simulink model "WindPrototipeN"  (R2019b)
settings: Solver=ode23s  StartTime=0.0  StopTime=Ts  FixedStep=2  RelTol=5
values from neighbouring files (symbols this model uses):
  c1 = 0.51763    [matlab.mat]
  c2 = 116    [matlab.mat]
  c3 = 0.4    [matlab.mat]
  c4 = 5    [matlab.mat]
  c5 = 21    [matlab.mat]
  c6 = 0.006795    [matlab.mat]
  Tp = 2e-05    [matlab.mat]
undefined symbols (not defined in the file or in its folder): Cogent, DiscIntNeverNeededParam, Ion, Kepware, Lithium, localhost, sigbuilder_block
libraries: powerlib x266, powerlib_extras x83, simulink x30, powerlib_meascontrol x13, opclib x11, sldrtlib x8, electricdrivelib x3
(part 5 of 9)

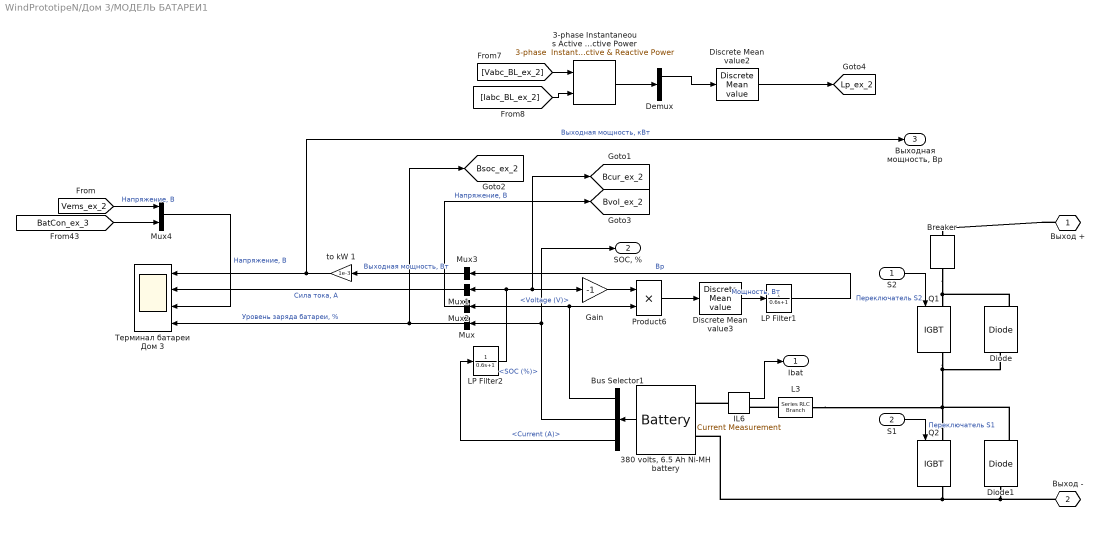
== system WindPrototipeN/Дом 3/МОДЕЛЬ БАТАРЕИ1 ==
  S2 : Inport
  S1 : Inport  Port=2
  3-phase Instantaneous Active & Reactive Power : powerlib_extras/Measurements/3-phase  Instantaneous  Active & Reactive Power
      settings: SourceProductName=Simscape Electrical  SourceProductBaseCode=PS
  "380 volts, 6.5 Ah Ni-MH battery " : electricdrivelib/Extra Sources/Battery  BatType=Lithium-Ion  ShowTempParam=off  ThermalPreset=no  ShowAgeParam=off  NomV=380  NomQ=2  SOC=56  Batt_Tr=10  PresetModel=on  MaxQ=2  MinV=285  FullV=442.3151  Dis_rate=0.86957  R=1.9  Normal_OP=1.8087  expZone="[410.5466    0.09826087]"  current=[6.5 13 32.5]  Units=Time  Tci=20  NomT=20  T2=-30  MaxQ2=4.8  FullV2=7.1  Normal_OP2=5.655  expZone2="[6.58           1]"  Rca=0.6  ti=2000  Dp=0  Neq0=0  Tsim=1e6  Ta1=25  Qeol=5.4*0.9  Reol=0.013333*1.2  Char_age=[2.3478, 3]  Dis_age=[2.3478, 10]  N1=1500  N2=10500  N3=1000  N4=1400  Ta2=45  N5=950
      settings: SourceProductName=Simscape Electrical
  Breaker : powerlib/Elements/Breaker  InitialState=1  SwitchingTimes=[15 ]  External=off  BreakerResistance=0.01  SnubberResistance=1e6  SnubberCapacitance=inf  Measurements=None  MoreParameters=off  NoBreakLoop=off
      settings: SourceProductName=Simscape Electrical
  Bus Selector1 : BusSelector  OutputSignals=Voltage (V),SOC (%),Current (A)
  Demux : Demux  Outputs=2
  Diode : powerlib/Power Electronics/Diode  Ron=0.001  Lon=0  Vf=0.8  IC=0  UseSnubber=off  Rs=500  Cs=250e-9  Measurements=on
      settings: SourceProductName=Simscape Electrical
  Diode1 : powerlib/Power Electronics/Diode  Ron=0.001  Lon=0  Vf=0.8  IC=0  UseSnubber=off  Rs=500  Cs=250e-9  Measurements=on
      settings: SourceProductName=Simscape Electrical
  Discrete Mean value2 : powerlib_extras/Discrete Measurements/Discrete  Mean value  Freq=50  Vinit=0  Ts=20e-6
      settings: SourceProductName=Simscape Electrical  SourceProductBaseCode=PS
  Discrete Mean value3 : powerlib_extras/Discrete Measurements/Discrete  Mean value  Freq=50  Vinit=0  Ts=20e-6
      settings: SourceProductName=Simscape Electrical  SourceProductBaseCode=PS
  Gain : Gain  Gain=-1
  IL6 : powerlib/Measurements/Current Measurement  PhasorSimulation=off  OutputType=Complex  PSBequivalent=0
      settings: SourceProductName=Simscape Electrical
  L3 : powerlib/Elements/Series RLC Branch  LConnTagsString=__new0  RConnTagsString=__new0  BranchType=L  Resistance=1.0  Inductance=5e-3  SetiL0=off  InitialCurrent=0  Capacitance=1.0  Setx0=off  InitialVoltage=0  Measurements=None
      settings: SourceProductName=Simscape Electrical
  LP Filter1 : TransferFcn  Denominator=[0.6 1]
  LP Filter2 : TransferFcn  Denominator=[0.6 1]
  Mux{,1..3} (4 alike) : Mux  Inputs=1
  Mux4 : Mux  Inputs=2
  Product6 : Product  RndMeth=Zero
  Q1 : powerlib/Power Electronics/IGBT  Ron=0.001  Lon=0  Vf=1  Tf=1e-6  Tt=2e-6  IC=0  Rs=1e5  Cs=inf  Measurements=on
      settings: SourceProductName=Simscape Electrical
  Q2 : powerlib/Power Electronics/IGBT  Ron=0.001  Lon=0  Vf=1  Tf=1e-6  Tt=2e-6  IC=0  Rs=1e5  Cs=inf  Measurements=on
      settings: SourceProductName=Simscape Electrical
  to kW 1 : Gain  Gain=1e-3
  Терминал батареи Дом 3 : Scope  NumInputPorts=4
  Выход + : PMIOPort  Tag=PMCPort  Side=Right
  " Выход -" : PMIOPort  Tag=PMCPort  Port=2  Side=Right
  Ibat : Outport  VectorParamsAs1DForOutWhenUnconnected=off
  "SOC, %" : Outport  Port=2  VectorParamsAs1DForOutWhenUnconnected=off
  "Выходная мощность, Bp" : Outport  Port=3  VectorParamsAs1DForOutWhenUnconnected=off
  tag scope: Bcur_ex_2=global, Bsoc_ex_2=global, Bvol_ex_2=global, Lp_ex_2=global
  wires:
  "380 volts, 6.5 Ah Ni-MH battery "/1 -> Bus Selector1/1
  Bus Selector1/1 -> Mux2/1, Product6/2  "<Voltage (V)>"
  Bus Selector1/2 -> Mux/1, "SOC, %"/1  "<SOC (%)>"
  Bus Selector1/3 -> LP Filter2/1  "<Current (A)>"
  S2/1 -> Q1/1  "Переключатель S2"
  S1/1 -> Q2/1  "Переключатель S1"
  IL6/1 -> Ibat/1
  Gain/1 -> Product6/1
  LP Filter2/1 -> Mux1/1, [Bcur_ex_2], Gain/1
  Discrete Mean value3/1 -> LP Filter1/1  "Мощность, Вт"
  Mux/1 -> [Bsoc_ex_2], Терминал батареи Дом 3/4  "Уровень заряда батареи, %"
  Mux1/1 -> Терминал батареи Дом 3/2  "Сила тока, А"
  Mux3/1 -> to kW 1/1  "Выходная мощность, Вт"
  Product6/1 -> Discrete Mean value3/1
  [Iabc_BL_ex_2] -> 3-phase Instantaneous Active & Reactive Power/2
  Discrete Mean value2/1 -> [Lp_ex_2]
  [Vabc_BL_ex_2] -> 3-phase Instantaneous Active & Reactive Power/1
  to kW 1/1 -> "Выходная мощность, Bp"/1, Терминал батареи Дом 3/1  "Выходная мощность, кВт"
  LP Filter1/1 -> Mux3/1  "Bp"
  Demux/1 -> Discrete Mean value2/1
  3-phase Instantaneous Active & Reactive Power/1 -> Demux/1
  Mux2/1 -> [Bvol_ex_2]  "Напряжение, В"
  [Vems_ex_2] -> Mux4/1  "Напряжение, В"
  Mux4/1 -> Терминал батареи Дом 3/3  "Напряжение, В"
  [BatCon_ex_3] -> Mux4/2
  connections:
  IL6/LConn1 -- "380 volts, 6.5 Ah Ni-MH battery "/LConn1
  Q2/RConn1 -- " Выход -"/RConn1 -- Diode1/LConn1 -- "380 volts, 6.5 Ah Ni-MH battery "/LConn2
  Выход +/RConn1 -- Breaker/LConn1
  Breaker/RConn1 -- Diode/RConn1 -- Q1/LConn1
  Q2/LConn1 -- Diode1/RConn1 -- Q1/RConn1 -- Diode/LConn1 -- L3/RConn1
  L3/LConn1 -- IL6/RConn1

== system WindPrototipeN/Дом 3/Мониторинг мощностей ==
  " to kW1" : Gain  Gain=1e-3
  Bus Creator1 : BusCreator  Inputs=4
  Discrete Mean value2 : powerlib_extras/Discrete Measurements/Discrete  Mean value  Freq=50  Vinit=0  Ts=20e-6
      settings: SourceProductName=Simscape Electrical  SourceProductBaseCode=PS
  Discrete Mean value3 : powerlib_extras/Discrete Measurements/Discrete  Mean value  Freq=50  Vinit=0  Ts=20e-6
      settings: SourceProductName=Simscape Electrical  SourceProductBaseCode=PS
  Discrete Mean value4 : powerlib_extras/Discrete Measurements/Discrete  Mean value  Freq=50  Vinit=0  Ts=20e-6
      settings: SourceProductName=Simscape Electrical  SourceProductBaseCode=PS
  "Power (3ph, Phasor)2" : powerlib_meascontrol/Measurements/Power (3ph, Phasor)
      settings: SourceProductName=Simscape Electrical  SourceProductBaseCode=PS
  Terminator2 : Terminator
  to kW 1 : Gain  Gain=1e-3
  to kW 2 : Gain  Gain=1e-3
  to kW 4 : Gain  Gain=1e-3
  Мощности Дом 3 : Scope
  wires:
  [Vload_ex_2] -> "Power (3ph, Phasor)2"/1
  [Lp_ex_2] -> to kW 1/1  "LP"
  [Wp_ex_2] -> Discrete Mean value4/1
  "Power (3ph, Phasor)2"/2 -> Terminator2/1
  Discrete Mean value2/1 -> " to kW1"/1
  to kW 2/1 -> Bus Creator1/3  "WP"
  to kW 4/1 -> Bus Creator1/2  "SP"
  " to kW1"/1 -> Bus Creator1/4  "Нагрузка"
  Discrete Mean value4/1 -> to kW 2/1
  [Iload_ex_2] -> "Power (3ph, Phasor)2"/2
  "Power (3ph, Phasor)2"/1 -> Discrete Mean value2/1
  Bus Creator1/1 -> Мощности Дом 3/1
  [Sp_ex_2] -> Discrete Mean value3/1
  Discrete Mean value3/1 -> to kW 4/1
  to kW 1/1 -> Bus Creator1/1  "Реактивная Б-Н"

== system WindPrototipeN/Дом 3/ПОТРЕБИТЕЛЬ1 ==
  1000 Вт1 : powerlib/Elements/Three-Phase Parallel RLC Load  LConnTagsString=A|B|C  Configuration=Y (grounded)  NominalVoltage=385  Vabc=[1e3 1e3 1e3]  Vabcp=[1e3 1e3 1e3]  NominalFrequency=50  UnbalancedPower=off  ActivePower=1000  InductivePower=0  CapacitivePower=0  Pabc=[10e3 9e3 11e3]  QLabc=[100 90 110]  QCabc=[100 90 110]  Pabcp=[10e3 9e3 11e3]  QLabcp=[100 90 110]  QCabcp=[100 90 110]  Measurements=None  LoadType=constant Z
      settings: SourceProductName=Simscape Electrical
  1500 Вт1 : powerlib/Elements/Three-Phase Parallel RLC Load  LConnTagsString=A|B|C  Configuration=Y (grounded)  NominalVoltage=385  Vabc=[1e3 1e3 1e3]  Vabcp=[1e3 1e3 1e3]  NominalFrequency=50  UnbalancedPower=off  ActivePower=1000  InductivePower=0  CapacitivePower=0  Pabc=[10e3 9e3 11e3]  QLabc=[100 90 110]  QCabc=[100 90 110]  Pabcp=[10e3 9e3 11e3]  QLabcp=[100 90 110]  QCabcp=[100 90 110]  Measurements=None  LoadType=constant Z
      settings: SourceProductName=Simscape Electrical
  500 Вт (1)1 : powerlib/Elements/Three-Phase Parallel RLC Load  LConnTagsString=A|B|C  Configuration=Y (grounded)  NominalVoltage=385  Vabc=[1e3 1e3 1e3]  Vabcp=[1e3 1e3 1e3]  NominalFrequency=50  UnbalancedPower=off  ActivePower=500  InductivePower=0  CapacitivePower=0  Pabc=[10e3 9e3 11e3]  QLabc=[100 90 110]  QCabc=[100 90 110]  Pabcp=[10e3 9e3 11e3]  QLabcp=[100 90 110]  QCabcp=[100 90 110]  Measurements=None  LoadType=constant Z
      settings: SourceProductName=Simscape Electrical
  500 Вт (2)1 : powerlib/Elements/Three-Phase Parallel RLC Load  LConnTagsString=A|B|C  Configuration=Y (grounded)  NominalVoltage=385  Vabc=[1e3 1e3 1e3]  Vabcp=[1e3 1e3 1e3]  NominalFrequency=50  UnbalancedPower=off  ActivePower=500  InductivePower=0  CapacitivePower=0  Pabc=[10e3 9e3 11e3]  QLabc=[100 90 110]  QCabc=[100 90 110]  Pabcp=[10e3 9e3 11e3]  QLabcp=[100 90 110]  QCabcp=[100 90 110]  Measurements=None  LoadType=constant Z
      settings: SourceProductName=Simscape Electrical
  BL : powerlib/Measurements/Three-Phase V-I Measurement  VoltageMeasurement=phase-to-ground  SetLabelV=on  LabelV=Vabc_BL_ex_2  Vpu=off  VpuLL=off  CurrentMeasurement=yes  SetLabelI=on  LabelI=Iabc_BL_ex_2  Ipu=off  Pbase=100e6  Vbase=500e3  OutputType=Magnitude  PhasorSimulation=off  PSBequivalent=0
      settings: SourceProductName=Simscape Electrical
  Subsystem1 : Subsystem
  Three-Phase Breaker10 : powerlib/Elements/Three-Phase Breaker  InitialState=open  SwitchA=on  SwitchB=on  SwitchC=on  SwitchTimes=[6 7]  External=on  BreakerResistance=0.001  SnubberResistance=1e6  SnubberCapacitance=inf  Measurements=None
      settings: SourceProductName=Simscape Electrical
  Three-Phase Breaker11 : powerlib/Elements/Three-Phase Breaker  InitialState=open  SwitchA=on  SwitchB=on  SwitchC=on  SwitchTimes=[7 10]  External=on  BreakerResistance=0.001  SnubberResistance=1e6  SnubberCapacitance=inf  Measurements=None
      settings: SourceProductName=Simscape Electrical
  Three-Phase Breaker8 : powerlib/Elements/Three-Phase Breaker  InitialState=open  SwitchA=on  SwitchB=on  SwitchC=on  SwitchTimes=[0 5]  External=on  BreakerResistance=0.001  SnubberResistance=1e6  SnubberCapacitance=inf  Measurements=None
      settings: SourceProductName=Simscape Electrical
  Three-Phase Breaker9 : powerlib/Elements/Three-Phase Breaker  InitialState=open  SwitchA=on  SwitchB=on  SwitchC=on  SwitchTimes=[2 5]  External=on  BreakerResistance=0.001  SnubberResistance=1e6  SnubberCapacitance=inf  Measurements=None
      settings: SourceProductName=Simscape Electrical
  Блок измерений : powerlib/Measurements/Three-Phase V-I Measurement  VoltageMeasurement=phase-to-ground  SetLabelV=off  LabelV=V1  Vpu=off  VpuLL=off  CurrentMeasurement=yes  SetLabelI=off  LabelI=I1  Ipu=off  Pbase=5.5e3  Vbase=385  OutputType=Magnitude  PhasorSimulation=off  PSBequivalent=0
      settings: SourceProductName=Simscape Electrical
  Терминал нагрузки : Scope  NumInputPorts=2
  A : PMIOPort  Side=Left
  B : PMIOPort  Port=2  Side=Left
  C : PMIOPort  Port=3  Side=Left
  tag scope: Iload_ex_2=global, Load3Home1=global, Load3Home2=global, Load3Home3=global, Load3Home4=global, Vload_ex_2=global
  wires:
  Блок измерений/1 -> [Vload_ex_2], Терминал нагрузки/1  "Напряжение, В"
  Блок измерений/2 -> [Iload_ex_2], Терминал нагрузки/2  "Сила тока, А"
  Subsystem1/1(Out1) -> [Load3Home1], Three-Phase Breaker8/1
  Subsystem1/4(Out4) -> [Load3Home4], Three-Phase Breaker11/1
  Subsystem1/3(Out3) -> [Load3Home3], Three-Phase Breaker10/1
  Subsystem1/2(Out2) -> [Load3Home2], Three-Phase Breaker9/1
  connections:
  BL/RConn1 -- Блок измерений/LConn1
  BL/RConn2 -- Блок измерений/LConn2
  BL/RConn3 -- Блок измерений/LConn3
  BL/LConn1 -- A/RConn1
  BL/LConn2 -- B/RConn1
  C/RConn1 -- BL/LConn3
  500 Вт (2)1/LConn3 -- Three-Phase Breaker9/LConn3
  500 Вт (2)1/LConn2 -- Three-Phase Breaker9/LConn2
  1500 Вт1/LConn1 -- Three-Phase Breaker11/LConn1
  1000 Вт1/LConn3 -- Three-Phase Breaker10/LConn3
  500 Вт (1)1/LConn2 -- Three-Phase Breaker8/LConn2
  1000 Вт1/LConn2 -- Three-Phase Breaker10/LConn2
  500 Вт (2)1/LConn1 -- Three-Phase Breaker9/LConn1
  500 Вт (1)1/LConn1 -- Three-Phase Breaker8/LConn1
  1000 Вт1/LConn1 -- Three-Phase Breaker10/LConn1
  500 Вт (1)1/LConn3 -- Three-Phase Breaker8/LConn3
  1500 Вт1/LConn3 -- Three-Phase Breaker11/LConn3
  1500 Вт1/LConn2 -- Three-Phase Breaker11/LConn2
  Блок измерений/RConn1 -- Three-Phase Breaker8/RConn1 -- Three-Phase Breaker9/RConn1 -- Three-Phase Breaker10/RConn1 -- Three-Phase Breaker11/RConn1
  Блок измерений/RConn2 -- Three-Phase Breaker8/RConn2 -- Three-Phase Breaker9/RConn2 -- Three-Phase Breaker10/RConn2 -- Three-Phase Breaker11/RConn2
  Блок измерений/RConn3 -- Three-Phase Breaker8/RConn3 -- Three-Phase Breaker9/RConn3 -- Three-Phase Breaker10/RConn3 -- Three-Phase Breaker11/RConn3

== system WindPrototipeN/Дом 3/СОЛНЕЧНЫЕ ПАНЕЛИ1 ==
  note: boost
  Солнечная радиация : Inport
  11*2=666 V : Subsystem
  FW Diode1 : powerlib/Power Electronics/Diode  Ron=0.01  Lon=0  Vf=0.8  IC=0  UseSnubber=off  Rs=100  Cs=0.1e-6  Measurements=off
      settings: SourceProductName=Simscape Electrical
  Gain : Gain  Gain=4732*2/1000
  IL1 : powerlib/Measurements/Current Measurement  PhasorSimulation=off  OutputType=Complex  PSBequivalent=0
      settings: SourceProductName=Simscape Electrical
  Mean Value1 : powerlib_extras/Measurements/Mean Value  Period=0.0045
      settings: SourceProductName=Simscape Electrical  SourceProductBaseCode=PS
  Mux : Mux  Inputs=2
  Product6 : Product  RndMeth=Zero
  Vdc2 : powerlib/Measurements/Voltage Measurement  Tag=PoWeRsYsTeMmEaSuReMeNt  PhasorSimulation=off  OutputType=Magnitude  PSBequivalent=0
      settings: SourceProductName=Simscape Electrical
  Мощность СП1 : Scope
  Мощность СП2 : Scope
  Мощность СП3_2 : Scope
  Мощность СП_2 : Scope
  Терминал данных параметров солнечной панели2 : Scope  NumInputPorts=4
  + : PMIOPort  Side=Right
  - : PMIOPort  Port=2  Side=Right
  Sp : Outport  VectorParamsAs1DForOutWhenUnconnected=off
  tag scope: Scur_ex_2=global, Sp_ex_2=global, Svol_ex_2=global
  wires:
  Vdc2/1 -> [Svol_ex_2], Мощность СП2/1, Терминал данных параметров солнечной панели2/4, Product6/1  "Напряжение, В"
  Product6/1 -> Mux/2, Sp/1, Терминал данных параметров солнечной панели2/2, [Sp_ex_2]  "Выходная мощность СЭУ, Вт"
  Gain/1 -> Mux/1, Терминал данных параметров солнечной панели2/1  "Интенсивность солнечной радиации, Вт/м2"
  Mux/1 -> Мощность СП_2/1
  Mean Value1/1 -> Product6/2
  IL1/1 -> [Scur_ex_2], Терминал данных параметров солнечной панели2/3, Mean Value1/1, Мощность СП1/1  "Сила тока, А"
  Солнечная радиация/1 -> Gain/1, Мощность СП3_2/1, 11*2=666 V/1(In1)
  connections:
  11*2=666 V/RConn2 -- Vdc2/LConn2 -- -/RConn1
  +/RConn1 -- IL1/RConn1
  11*2=666 V/RConn1 -- FW Diode1/LConn1 -- Vdc2/LConn1
  IL1/LConn1 -- FW Diode1/RConn1

== system WindPrototipeN/СИСТЕМА EMS/Chart3/ESS.LoadDispatcherMode.powerman ==
  Vbat_cmd : Inport  OutDataTypeStr=double  PortDimensions=1
  Bpower : Inport  Port=2  OutDataTypeStr=double  PortDimensions=1
  f : TriggerPort  TriggerType=function-call  VariantControl=(inherit)
      settings: CopyFcn=Stateflow.SLINSF.SimulinkMan.removeBlockPreDeleteFcn  PreDeleteFcn=Stateflow.SLINSF.SimulinkMan.unsafePredeleteFcn
  Chart : Stateflow chart  BlockKeywords=__PRM__SERIALIZED__DATA__:Stateflow Chart,Stateflow Diagram  TreatAsAtomicUnit=on
  y : Outport
  wires:
  Chart/1(VoltageRef) -> y/1
  Vbat_cmd/1 -> Chart/2(Vbatcmd)
  Bpower/1 -> Chart/1(Bp)

== system WindPrototipeN/СИСТЕМА EMS/EMS дом 1/ESS.LoadDispatcherMode.powerman ==
  Vbat_cmd : Inport  OutDataTypeStr=double  PortDimensions=1
  Bpower : Inport  Port=2  OutDataTypeStr=double  PortDimensions=1
  f : TriggerPort  TriggerType=function-call  VariantControl=(inherit)
      settings: CopyFcn=Stateflow.SLINSF.SimulinkMan.removeBlockPreDeleteFcn  PreDeleteFcn=Stateflow.SLINSF.SimulinkMan.unsafePredeleteFcn
  Chart : Stateflow chart  BlockKeywords=__PRM__SERIALIZED__DATA__:Stateflow Chart,Stateflow Diagram  TreatAsAtomicUnit=on
  y : Outport
  wires:
  Chart/1(VoltageRef) -> y/1
  Vbat_cmd/1 -> Chart/2(Vbatcmd)
  Bpower/1 -> Chart/1(Bp)

== system WindPrototipeN/СИСТЕМА EMS/EMS дом 2/ESS.LoadDispatcherMode.powerman ==
  Vbat_cmd : Inport  OutDataTypeStr=double  PortDimensions=1
  Bpower : Inport  Port=2  OutDataTypeStr=double  PortDimensions=1
  f : TriggerPort  TriggerType=function-call  VariantControl=(inherit)
      settings: CopyFcn=Stateflow.SLINSF.SimulinkMan.removeBlockPreDeleteFcn  PreDeleteFcn=Stateflow.SLINSF.SimulinkMan.unsafePredeleteFcn
  Chart : Stateflow chart  BlockKeywords=__PRM__SERIALIZED__DATA__:Stateflow Chart,Stateflow Diagram  TreatAsAtomicUnit=on
  y : Outport
  wires:
  Chart/1(VoltageRef) -> y/1
  Vbat_cmd/1 -> Chart/2(Vbatcmd)
  Bpower/1 -> Chart/1(Bp)

== system WindPrototipeN/СИСТЕМА EMS/EMS дом 3/ESS.LoadDispatcherMode.powerman ==
  Vbat_cmd : Inport  OutDataTypeStr=double  PortDimensions=1
  Bpower : Inport  Port=2  OutDataTypeStr=double  PortDimensions=1
  f : TriggerPort  TriggerType=function-call  VariantControl=(inherit)
      settings: CopyFcn=Stateflow.SLINSF.SimulinkMan.removeBlockPreDeleteFcn  PreDeleteFcn=Stateflow.SLINSF.SimulinkMan.unsafePredeleteFcn
  Chart : Stateflow chart  BlockKeywords=__PRM__SERIALIZED__DATA__:Stateflow Chart,Stateflow Diagram  TreatAsAtomicUnit=on
  y : Outport
  wires:
  Chart/1(VoltageRef) -> y/1
  Vbat_cmd/1 -> Chart/2(Vbatcmd)
  Bpower/1 -> Chart/1(Bp)

== system WindPrototipeN/СИСТЕМА EMS/OPC ==
  In1 : Inport
  In2 : Inport  Port=2
  In3 : Inport  Port=3
  Demux : Demux  Outputs=3
  Mux : Mux  Inputs=3
  OPC Configuration : opclib/OPC Configuration  opcServers=localhost/Kepware.KEPServerEX.V6/1, localhost/Cogent.DataHub.1/5.000000e-01  errMissingItems=Error  errReadWrite=Warn  errShutdown=Error  errRTViolation=Warn  rtEnable=on  speedup=60  showLatency=off  beingUsed=on
      settings: SourceProductName=OPC Toolbox  SourceProductBaseCode=OT
  OPC Read : opclib/OPC Read  serverHost=localhost  serverID=Kepware.KEPServerEX.V6  itemIDs=Channel1.Device1.PpostHome1, Channel1.Device1.PpostHome2, Channel1.Device1.PpostHome3  readMode=Asynchronous (device)  dataType=int32  updateRate=0.05  showQual=off  showTS=off  tsMode=Seconds since start
      settings: SourceProductName=OPC Toolbox  SourceProductBaseCode=OT
  OPC Write : opclib/OPC Write  serverHost=localhost  serverID=Kepware.KEPServerEX.V6  itemIDs=Channel1.Device1.PpostHome1, Channel1.Device1.PpostHome2, Channel1.Device1.PpostHome3  writeMode=Synchronous  updateRate=0.05
      settings: SourceProductName=OPC Toolbox  SourceProductBaseCode=OT
  Subsystem : Subsystem
  Out1 : Outport
  Out2 : Outport  Port=2
  Out3 : Outport  Port=3
  wires:
  Subsystem/1(Out1) -> Out1/1
  In1/1 -> Mux/1
  Subsystem/3(Out3) -> Out3/1
  Demux/2 -> Subsystem/2(In2)
  Demux/3 -> Subsystem/3(In3)
  Mux/1 -> OPC Write/1
  OPC Read/1 -> Demux/1
  Demux/1 -> Subsystem/1(In1)
  Subsystem/2(Out2) -> Out2/1
  In3/1 -> Mux/3
  In2/1 -> Mux/2

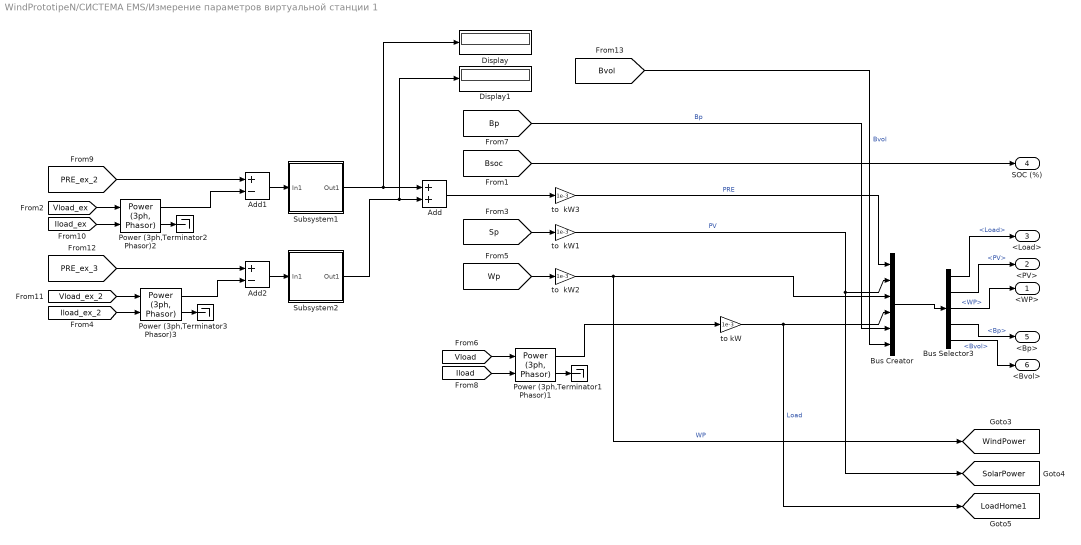
== system WindPrototipeN/СИСТЕМА EMS/Измерение параметров виртуальной станции 1 ==
  " to kW" : Gain  Gain=1e-3
  Add : Sum
  Add1 : Sum  Inputs=+-
  Add2 : Sum  Inputs=+-
  Bus Creator : BusCreator  Inputs=6
  Bus Selector3 : BusSelector  OutputSignals=Load,PV,WP,Bp,Bvol
  Display : Display
  Display1 : Display
  "Power (3ph, Phasor)1" : powerlib_meascontrol/Measurements/Power (3ph, Phasor)
      settings: SourceProductName=Simscape Electrical  SourceProductBaseCode=PS
  "Power (3ph, Phasor)2" : powerlib_meascontrol/Measurements/Power (3ph, Phasor)
      settings: SourceProductName=Simscape Electrical  SourceProductBaseCode=PS
  "Power (3ph, Phasor)3" : powerlib_meascontrol/Measurements/Power (3ph, Phasor)
      settings: SourceProductName=Simscape Electrical  SourceProductBaseCode=PS
  Subsystem1 : Subsystem
  Subsystem2 : Subsystem
  Terminator1 : Terminator
  Terminator2 : Terminator
  Terminator3 : Terminator
  to  kW1 : Gain  Gain=1e-3
  to  kW2 : Gain  Gain=1e-3
  to  kW3 : Gain  Gain=1e-3
  <WP> : Outport  VectorParamsAs1DForOutWhenUnconnected=off
  <PV> : Outport  Port=2  VectorParamsAs1DForOutWhenUnconnected=off
  <Load> : Outport  Port=3  VectorParamsAs1DForOutWhenUnconnected=off
  SOC (%) : Outport  Port=4  VectorParamsAs1DForOutWhenUnconnected=off
  <Bp> : Outport  Port=5  VectorParamsAs1DForOutWhenUnconnected=off
  <Bvol> : Outport  Port=6  VectorParamsAs1DForOutWhenUnconnected=off
  tag scope: LoadHome1=global, SolarPower=global, WindPower=global
  wires:
  Bus Creator/1 -> Bus Selector3/1
  "Power (3ph, Phasor)1"/2 -> Terminator1/1
  " to kW"/1 -> [LoadHome1], Bus Creator/4  "Load"
  [Vload] -> "Power (3ph, Phasor)1"/1
  [Iload] -> "Power (3ph, Phasor)1"/2
  "Power (3ph, Phasor)1"/1 -> " to kW"/1
  Bus Selector3/2 -> <PV>/1  "<PV>"
  Bus Selector3/1 -> <Load>/1  "<Load>"
  [Bsoc] -> SOC (%)/1
  to  kW1/1 -> Bus Creator/2, [SolarPower]  "PV"
  to  kW2/1 -> [WindPower], Bus Creator/3  "WP"
  Bus Selector3/3 -> <WP>/1  "<WP>"
  [Sp] -> to  kW1/1
  [Wp] -> to  kW2/1
  Add/1 -> to  kW3/1
  [PRE_ex_2] -> Add1/1
  "Power (3ph, Phasor)2"/2 -> Terminator2/1
  [Iload_ex] -> "Power (3ph, Phasor)2"/2
  "Power (3ph, Phasor)2"/1 -> Add1/2
  [Vload_ex] -> "Power (3ph, Phasor)2"/1
  "Power (3ph, Phasor)3"/2 -> Terminator3/1
  "Power (3ph, Phasor)3"/1 -> Add2/2
  [PRE_ex_3] -> Add2/1
  [Iload_ex_2] -> "Power (3ph, Phasor)3"/2
  [Vload_ex_2] -> "Power (3ph, Phasor)3"/1
  Add2/1 -> Subsystem2/1(In1)
  Add1/1 -> Subsystem1/1(In1)
  Subsystem1/1(Out1) -> Display/1, Add/1
  Subsystem2/1(Out1) -> Add/2, Display1/1
  to  kW3/1 -> Bus Creator/1  "PRE"
  [Bp] -> Bus Creator/5  "Bp"
  Bus Selector3/4 -> <Bp>/1  "<Bp>"
  [Bvol] -> Bus Creator/6  "Bvol"
  Bus Selector3/5 -> <Bvol>/1  "<Bvol>"

== system WindPrototipeN/СИСТЕМА EMS/станция 2 ==
  " to kW" : Gain  Gain=1e-3
  Add : Sum
  Add1 : Sum  Inputs=+-
  Add2 : Sum  Inputs=+-
  Bus Creator1 : BusCreator  Inputs=6
  Bus Selector1 : BusSelector  OutputSignals=Load,PV,WP,Bp,Bvol
  Display : Display
  Display1 : Display
  "Power (3ph, Phasor)1" : powerlib_meascontrol/Measurements/Power (3ph, Phasor)
      settings: SourceProductName=Simscape Electrical  SourceProductBaseCode=PS
  "Power (3ph, Phasor)2" : powerlib_meascontrol/Measurements/Power (3ph, Phasor)
      settings: SourceProductName=Simscape Electrical  SourceProductBaseCode=PS
  "Power (3ph, Phasor)3" : powerlib_meascontrol/Measurements/Power (3ph, Phasor)
      settings: SourceProductName=Simscape Electrical  SourceProductBaseCode=PS
  Subsystem1 : Subsystem
  Subsystem2 : Subsystem
  Terminator1 : Terminator
  Terminator2 : Terminator
  Terminator3 : Terminator
  to  kW1 : Gain  Gain=1e-3
  to  kW2 : Gain  Gain=1e-3
  to  kW3 : Gain  Gain=1e-3
  <WP> : Outport  VectorParamsAs1DForOutWhenUnconnected=off
  <PV> : Outport  Port=2  VectorParamsAs1DForOutWhenUnconnected=off
  <Load> : Outport  Port=3  VectorParamsAs1DForOutWhenUnconnected=off
  SOC (%) : Outport  Port=4  VectorParamsAs1DForOutWhenUnconnected=off
  <Bp> : Outport  Port=5  VectorParamsAs1DForOutWhenUnconnected=off
  <Bvol> : Outport  Port=6  VectorParamsAs1DForOutWhenUnconnected=off
  tag scope: LoadHome2=global
  wires:
  "Power (3ph, Phasor)1"/2 -> Terminator1/1
  " to kW"/1 -> [LoadHome2], Bus Creator1/4  "Load"
  [Vload_ex] -> "Power (3ph, Phasor)1"/1
  [Iload_ex] -> "Power (3ph, Phasor)1"/2
  "Power (3ph, Phasor)1"/1 -> " to kW"/1
  [Bsoc_ex] -> SOC (%)/1
  to  kW1/1 -> Bus Creator1/1  "PV"
  to  kW2/1 -> Bus Creator1/5  "WP"
  [Sp_ex] -> to  kW1/1
  [Wp_ex] -> to  kW2/1
  to  kW3/1 -> Bus Creator1/3  "PRE"
  Add/1 -> to  kW3/1
  "Power (3ph, Phasor)3"/1 -> Add2/2
  [PRE_ex_3] -> Add2/1
  [Iload_ex_2] -> "Power (3ph, Phasor)3"/2
  "Power (3ph, Phasor)3"/2 -> Terminator3/1
  "Power (3ph, Phasor)2"/2 -> Terminator2/1
  "Power (3ph, Phasor)2"/1 -> Add1/2
  [PRE_ex_1] -> Add1/1
  [Vload] -> "Power (3ph, Phasor)2"/1
  [Iload] -> "Power (3ph, Phasor)2"/2
  [Vload_ex_2] -> "Power (3ph, Phasor)3"/1
  Add2/1 -> Subsystem2/1(In1)
  Add1/1 -> Subsystem1/1(In1)
  Subsystem1/1(Out1) -> Display/1, Add/1
  Subsystem2/1(Out1) -> Display1/1, Add/2
  [Bp_ex] -> Bus Creator1/2  "Bp"
  Bus Selector1/4 -> <Bp>/1  "<Bp>"
  Bus Creator1/1 -> Bus Selector1/1
  Bus Selector1/1 -> <Load>/1  "<Load>"
  Bus Selector1/2 -> <PV>/1  "<PV>"
  Bus Selector1/5 -> <Bvol>/1  "<Bvol>"
  [Bvol_ex] -> Bus Creator1/6  "Bvol"
  Bus Selector1/3 -> <WP>/1  "<WP>"

== system WindPrototipeN/СИСТЕМА EMS/станция 3 ==
  " to kW" : Gain  Gain=1e-3
  Add : Sum
  Add1 : Sum  Inputs=+-
  Add2 : Sum  Inputs=+-
  Bus Creator : BusCreator  Inputs=6
  Bus Selector3 : BusSelector  OutputSignals=WP,PV,Load,Bp,Bvol
  Display : Display
  Display1 : Display
  "Power (3ph, Phasor)1" : powerlib_meascontrol/Measurements/Power (3ph, Phasor)
      settings: SourceProductName=Simscape Electrical  SourceProductBaseCode=PS
  "Power (3ph, Phasor)2" : powerlib_meascontrol/Measurements/Power (3ph, Phasor)
      settings: SourceProductName=Simscape Electrical  SourceProductBaseCode=PS
  "Power (3ph, Phasor)3" : powerlib_meascontrol/Measurements/Power (3ph, Phasor)
      settings: SourceProductName=Simscape Electrical  SourceProductBaseCode=PS
  Subsystem1 : Subsystem
  Subsystem2 : Subsystem
  Terminator1 : Terminator
  Terminator2 : Terminator
  Terminator3 : Terminator
  to  kW1 : Gain  Gain=1e-3
  to  kW2 : Gain  Gain=1e-3
  to  kW3 : Gain  Gain=1e-3
  <WP> : Outport  VectorParamsAs1DForOutWhenUnconnected=off
  <PV> : Outport  Port=2  VectorParamsAs1DForOutWhenUnconnected=off
  <Load> : Outport  Port=3  VectorParamsAs1DForOutWhenUnconnected=off
  SOC (%) : Outport  Port=4  VectorParamsAs1DForOutWhenUnconnected=off
  <Bp> : Outport  Port=5  VectorParamsAs1DForOutWhenUnconnected=off
  <Bvol> : Outport  Port=6  VectorParamsAs1DForOutWhenUnconnected=off
  tag scope: LoadHome3=global
  wires:
  Bus Creator/1 -> Bus Selector3/1
  "Power (3ph, Phasor)1"/2 -> Terminator1/1
  " to kW"/1 -> [LoadHome3], Bus Creator/4  "Load"
  [Vload_ex_2] -> "Power (3ph, Phasor)1"/1
  [Iload_ex_2] -> "Power (3ph, Phasor)1"/2
  "Power (3ph, Phasor)1"/1 -> " to kW"/1
  [Bsoc_ex_2] -> SOC (%)/1
  to  kW1/1 -> Bus Creator/1  "PV"
  to  kW2/1 -> Bus Creator/5  "WP"
  [Sp_ex_2] -> to  kW1/1
  [Wp_ex_2] -> to  kW2/1
  to  kW3/1 -> Bus Creator/3  "PRE"
  Add/1 -> to  kW3/1
  "Power (3ph, Phasor)3"/1 -> Add2/2
  [PRE_ex_1] -> Add2/1
  [Iload] -> "Power (3ph, Phasor)3"/2
  "Power (3ph, Phasor)3"/2 -> Terminator3/1
  "Power (3ph, Phasor)2"/2 -> Terminator2/1
  "Power (3ph, Phasor)2"/1 -> Add1/2
  [PRE_ex_2] -> Add1/1
  [Vload_ex] -> "Power (3ph, Phasor)2"/1
  [Iload_ex] -> "Power (3ph, Phasor)2"/2
  [Vload] -> "Power (3ph, Phasor)3"/1
  Add1/1 -> Subsystem1/1(In1)
  Add2/1 -> Subsystem2/1(In1)
  Subsystem1/1(Out1) -> Display/1, Add/1
  Subsystem2/1(Out1) -> Display1/1, Add/2
  [Bp_ex_2] -> Bus Creator/2  "Bp"
  [Bvol_ex_2] -> Bus Creator/6  "Bvol"
  Bus Selector3/1 -> <WP>/1  "<WP>"
  Bus Selector3/2 -> <PV>/1  "<PV>"
  Bus Selector3/3 -> <Load>/1  "<Load>"
  Bus Selector3/4 -> <Bp>/1  "<Bp>"
  Bus Selector3/5 -> <Bvol>/1  "<Bvol>"

== system WindPrototipeN/SCADA DEMS/OPC/OPC дом 1 ==
  Mux : Mux  Inputs=24
  OPC Write1 : opclib/OPC Write  serverHost=localhost  serverID=Kepware.KEPServerEX.V6  itemIDs=Channel1.Device1.Home1.BatteryCurrent, Channel1.Device1.Home1.BatteryPower, Channel1.Device1.Home1.BatterySOC, Channel1.Device1.Home1.BatteryVoltage, Channel1.Device1.Home1.GridCurrent, Channel1.Device1.Home1.GridVoltage, Channel1.Device1.Home1.LoadPower, Channel1.Device1.Home1.SolarCurrent, Channel1.Device1.Home1.SolarPower, Channel1.Device1.Home1.SolarRad, Channel1.Device1.Home1.SolarVoltage, Channel1.Device1.Home1.WindSpeed, Channel1.Device1.Home1.WindTurbinePower, Channel1.Device1.Home1.WindTurbineVoltage, Channel1.Device1.Home1.WindTurbineCurrent, Channel1.Device1.Home1.WTDCcur, Channel1.Device1.Home1.WTDCvol, Channel1.Device1.Home1.SPDCcur, Channel1.Device1.Home1.SPDCvol, Channel1.Device1.Home1.Lp, Channel1.Device1.Home1.LoadCon, Channel1.Device1.Home1.BatRef, Channel1.Device1.Home1.Poutcmd, Channel1.Device1.Home1.Pincmd  writeMode=Synchronous  updateRate=0.05
      settings: SourceProductName=OPC Toolbox  SourceProductBaseCode=OT
  to  kW1 : Gain  Gain=1e-3
  to  kW3 : Gain  Gain=1e-3
  to  kW8 : Gain  Gain=1e-3
  wires:
  [Bvol] -> Mux/4
  [Wcur] -> Mux/15
  [Vems] -> Mux/6
  [Bsoc] -> Mux/3
  [Pin_ex_1] -> Mux/24
  [Wp] -> to  kW3/1
  to  kW8/1 -> Mux/20
  [Sp] -> to  kW1/1
  [Bp] -> Mux/2
  [Iems] -> Mux/5
  [Svol] -> Mux/11
  [SolarDCoutV] -> Mux/19
  [WindDCoutA] -> Mux/16
  [SolarRad] -> Mux/10
  to  kW3/1 -> Mux/13
  [SolarDCoutA] -> Mux/18
  [Wvol] -> Mux/14
  [LoadHome1] -> Mux/7
  [Pout_ex_1] -> Mux/23
  [BatCon_ex_1] -> Mux/22
  Mux/1 -> OPC Write1/1
  [ConLoad_ex_1] -> Mux/21
  [Lp] -> to  kW8/1
  [WindDCoutV] -> Mux/17
  to  kW1/1 -> Mux/9
  [Scur] -> Mux/8
  [Bcur] -> Mux/1
  [WindSpeed] -> Mux/12

== system WindPrototipeN/SCADA DEMS/OPC/OPC дом 2 ==
  Mux1 : Mux  Inputs=24
  OPC Write2 : opclib/OPC Write  serverHost=localhost  serverID=Kepware.KEPServerEX.V6  itemIDs=Channel1.Device1.Home2.BatteryCurrent, Channel1.Device1.Home2.BatteryPower, Channel1.Device1.Home2.BatterySOC, Channel1.Device1.Home2.BatteryVoltage, Channel1.Device1.Home2.GridCurrent, Channel1.Device1.Home2.GridVoltage, Channel1.Device1.Home2.LoadPower, Channel1.Device1.Home2.SolarCurrent, Channel1.Device1.Home2.SolarPower, Channel1.Device1.Home2.SolarRad, Channel1.Device1.Home2.SolarVoltage, Channel1.Device1.Home2.WindSpeed, Channel1.Device1.Home2.WindTurbinePower, Channel1.Device1.Home2.WindTurbineVoltage, Channel1.Device1.Home2.WindTurbineCurrent, Channel1.Device1.Home2.WTDCcur, Channel1.Device1.Home2.WTDCvol, Channel1.Device1.Home2.SPDCcur, Channel1.Device1.Home2.SPDCvol, Channel1.Device1.Home2.Lp, Channel1.Device1.Home2.LoadCon, Channel1.Device1.Home2.BatRef, Channel1.Device1.Home2.Poutcmd, Channel1.Device1.Home2.Pincmd  writeMode=Synchronous  updateRate=0.05
      settings: SourceProductName=OPC Toolbox  SourceProductBaseCode=OT
  to  kW2 : Gain  Gain=1e-3
  to  kW4 : Gain  Gain=1e-3
  to  kW9 : Gain  Gain=1e-3
  wires:
  [Lp_ex] -> to  kW9/1
  [ConLoad_ex_2] -> Mux1/21
  [Bcur_ex] -> Mux1/1
  [Bsoc_ex] -> Mux1/3
  [Iems_ex] -> Mux1/5
  [Wvol_ex] -> Mux1/14
  [WindDCoutA_ex] -> Mux1/16
  [BatCon_ex_2] -> Mux1/22
  [SolarRad_ex] -> Mux1/10
  [Pout_ex_2] -> Mux1/23
  [LoadHome2] -> Mux1/7
  [SolarDCoutA_ex] -> Mux1/18
  [WindDCoutV_ex] -> Mux1/17
  [Pin_ex_2] -> Mux1/24
  [Bp_ex] -> Mux1/2
  Mux1/1 -> OPC Write2/1
  [WindSpeed_ex] -> Mux1/12
  to  kW9/1 -> Mux1/20
  [Sp_ex] -> to  kW2/1
  [Vems_ex] -> Mux1/6
  to  kW2/1 -> Mux1/9
  [Scur_ex] -> Mux1/8
  [Svol_ex] -> Mux1/11
  [Wp_ex] -> to  kW4/1
  [SolarDCoutV_ex] -> Mux1/19
  [Bvol_ex] -> Mux1/4
  to  kW4/1 -> Mux1/13
  [Wcur_ex] -> Mux1/15

== system WindPrototipeN/SCADA DEMS/OPC/OPC дом 3 ==
  Mux2 : Mux  Inputs=24
  OPC Write3 : opclib/OPC Write  serverHost=localhost  serverID=Kepware.KEPServerEX.V6  itemIDs=Channel1.Device1.Home3.BatteryCurrent, Channel1.Device1.Home3.BatteryPower, Channel1.Device1.Home3.BatterySOC, Channel1.Device1.Home3.BatteryVoltage, Channel1.Device1.Home3.GridCurrent, Channel1.Device1.Home3.GridVoltage, Channel1.Device1.Home3.LoadPower, Channel1.Device1.Home3.SolarCurrent, Channel1.Device1.Home3.SolarPower, Channel1.Device1.Home3.SolarRad, Channel1.Device1.Home3.SolarVoltage, Channel1.Device1.Home3.WindSpeed, Channel1.Device1.Home3.WindTurbinePower, Channel1.Device1.Home3.WindTurbineVoltage, Channel1.Device1.Home3.WindTurbineCurrent, Channel1.Device1.Home3.WTDCcur, Channel1.Device1.Home3.WTDCvol, Channel1.Device1.Home3.SPDCcur, Channel1.Device1.Home3.SPDCvol, Channel1.Device1.Home3.Lp, Channel1.Device1.Home3.LoadCon, Channel1.Device1.Home3.BatRef, Channel1.Device1.Home3.Poutcmd, Channel1.Device1.Home3.Pincmd  writeMode=Synchronous  updateRate=0.05
      settings: SourceProductName=OPC Toolbox  SourceProductBaseCode=OT
  to  kW10 : Gain  Gain=1e-3
  to  kW5 : Gain  Gain=1e-3
  to  kW6 : Gain  Gain=1e-3
  wires:
  [Pin_ex_3] -> Mux2/24
  [Pout_ex_3] -> Mux2/23
  [Bsoc_ex_2] -> Mux2/3
  [Vems_ex_2] -> Mux2/6
  [SolarRad_ex_2] -> Mux2/10
  [BatCon_ex_3] -> Mux2/22
  [Wvol_ex_2] -> Mux2/14
  [Bp_ex_2] -> Mux2/2
  [Iems_ex_2] -> Mux2/5
  [Wp_ex_2] -> to  kW6/1
  Mux2/1 -> OPC Write3/1
  [Bcur_ex_2] -> Mux2/1
  to  kW6/1 -> Mux2/13
  [ConLoad_ex_3] -> Mux2/21
  [WindDCoutA_ex_2] -> Mux2/16
  [SolarDCoutA_ex_2] -> Mux2/18
  [Svol_ex_2] -> Mux2/11
  [WindSpeed_ex_2] -> Mux2/12
  [LoadHome3] -> Mux2/7
  [SolarDCoutV_ex_2] -> Mux2/19
  [WindDCoutV_ex_2] -> Mux2/17
  to  kW5/1 -> Mux2/9
  [Bvol_ex_2] -> Mux2/4
  to  kW10/1 -> Mux2/20
  [Sp_ex_2] -> to  kW5/1
  [Wcur_ex_2] -> Mux2/15
  [Lp_ex_2] -> to  kW10/1
  [Scur_ex_2] -> Mux2/8

== system WindPrototipeN/SCADA DEMS/OPC/OPC прочее ==
  Data Type Conversion : DataTypeConversion  OutDataTypeStr=int8
  Mux3 : Mux  Inputs=12
  OPC Write4 : opclib/OPC Write  serverHost=localhost  serverID=Kepware.KEPServerEX.V6  itemIDs=Channel1.Device1.HouseConsumption.Home1Load1, Channel1.Device1.HouseConsumption.Home1Load2, Channel1.Device1.HouseConsumption.Home1Load3, Channel1.Device1.HouseConsumption.Home1Load4, Channel1.Device1.HouseConsumption.Home2Load1, Channel1.Device1.HouseConsumption.Home2Load2, Channel1.Device1.HouseConsumption.Home2Load3, Channel1.Device1.HouseConsumption.Home2Load4, Channel1.Device1.HouseConsumption.Home3Load1, Channel1.Device1.HouseConsumption.Home3Load2, Channel1.Device1.HouseConsumption.Home3Load3, Channel1.Device1.HouseConsumption.Home3Load4  writeMode=Synchronous  updateRate=0.05
      settings: SourceProductName=OPC Toolbox  SourceProductBaseCode=OT
  wires:
  [Load2Home1] -> Mux3/5
  [Load3Home4] -> Mux3/12
  [Load3Home3] -> Mux3/11
  [Load1Home4] -> Mux3/4
  [Load1Home1] -> Mux3/1
  [Load3Home1] -> Mux3/9
  [Load2Home4] -> Mux3/8
  [Load2Home2] -> Mux3/6
  [Load1Home2] -> Mux3/2
  [Load1Home3] -> Mux3/3
  [Load3Home2] -> Mux3/10
  Data Type Conversion/1 -> OPC Write4/1
  [Load2Home3] -> Mux3/7
  Mux3/1 -> Data Type Conversion/1

== system WindPrototipeN/Дом 1/DC//AC 220В/LC Фильтр ==
  "2 mH " : powerlib/Elements/Three-Phase Series RLC Branch  LConnTagsString=A|B|C  RConnTagsString=A|B|C  BranchType=L  Resistance=1.0  Inductance=36e-4  Capacitance=1.0  Measurements=None
      settings: SourceProductName=Simscape Electrical
  Ground : powerlib/Elements/Ground  LConnTagsString=a
      settings: SourceProductName=Simscape Electrical
  Ground1 : powerlib/Elements/Ground  LConnTagsString=a
      settings: SourceProductName=Simscape Electrical
  Ground2 : powerlib/Elements/Ground  LConnTagsString=a
      settings: SourceProductName=Simscape Electrical
  Three-Phase Series RLC Branch : powerlib/Elements/Three-Phase Series RLC Branch  LConnTagsString=A|B|C  RConnTagsString=A|B|C  BranchType=C  Resistance=.1  Inductance=1e-3  Capacitance=6.85e-6  Measurements=None
      settings: SourceProductName=Simscape Electrical
  A : PMIOPort  Side=Left
  B : PMIOPort  Port=2  Side=Left
  C : PMIOPort  Port=3  Side=Left
  "A " : PMIOPort  Port=4  Side=Right
  "B " : PMIOPort  Port=5  Side=Right
  "C " : PMIOPort  Port=6  Side=Right
  connections:
  B/RConn1 -- "2 mH "/LConn2
  A/RConn1 -- "2 mH "/LConn1
  C/RConn1 -- "2 mH "/LConn3
  "2 mH "/RConn1 -- "A "/RConn1 -- Three-Phase Series RLC Branch/LConn1
  "2 mH "/RConn2 -- "B "/RConn1 -- Three-Phase Series RLC Branch/LConn2
  "2 mH "/RConn3 -- "C "/RConn1 -- Three-Phase Series RLC Branch/LConn3
  Ground/LConn1 -- Three-Phase Series RLC Branch/RConn1
  Ground1/LConn1 -- Three-Phase Series RLC Branch/RConn2
  Ground2/LConn1 -- Three-Phase Series RLC Branch/RConn3

== system WindPrototipeN/Дом 1/DC//AC 220В/Инвертор DC//AC ==
  Discrete PWM Generator1 : Subsystem  AncestorBlock=|  DialogController=POWERSYS.PowerSysDialog  mask(Discrete PWM Generator){GeneratorMode=3-arm  bridge (6 pulses), Fc=4000, Ts=20e-6, Internal=off, mIndex=0.4, Freq=60, Phase=0}
      | powerlib_extras/Discrete 
      | Control Blocks/Discrete
      | PWM Generator
      mask prompts: GeneratorMode "Generator Mode"; Fc "Carrier frequency (Hz):"; Ts "Sample time:"; Internal "Internal generation of modulating signal(s)"; mIndex "Modulation index  (0<m<1) :"; Freq "Frequency of output voltage (Hz)"; Phase "Phase of output voltage (degrees)"
      mask help:
      | This discrete block generates pulses for carrier-based PWM (Pulse Width Modulation), self-commutated IGBTs,GTOs or FETs bridges.
      |
      | Depending on the number of bridge arms selected in the "Generator Mode" parameter, the block can be used either for single-phase or three-phase PWM control.
      mask init:
      | powericon('psbcallbacks',gcb,'Discrete PWM Generator');
      | if Freq==0
      |     Phase=90;
      | end
      | switch GeneratorMode
      | case 1,
      |     Internal_Phase=0;
      |    Signal_PortWidth=1;
      |    Select1_Elements=[1 2];
      |    Select1_PortWidth=2;
      |    Select3_Elements=[1 2];
      |    Select3_PortWidth=4;
      | case 2,
      |     Internal_Phase=0;
      |     Signal_PortWidth=1;
      |     Select1_Elements=[1 2];
      |     Select1_PortWidth=2;
      |     Select3_Elements=[1 2 3 4];
      |     Select3_PortWidth=4;
      | case 3,
      |     Internal_Phase=[0 -2*pi/3 2*pi/3];
      |     Signal_PortWidth=3;
      |     Select1_Elements=[1 4 2 5 3 6];
      |     Select1_PortWidth=6;
      |    Select3_Elements=[1 2 3 4 5 6];
      |    Select3_PortWidth=12;
      | case 4,
      |     Internal_Phase=[0 -2*pi/3 2*pi/3];
      |     Signal_PortWidth=3;
      |     Select1_Elements=[1 4 2 5 3 6];
      |     Select1_PortWidth=6;
      |    Select3_Elements=[1 2 3 4 5 6 7 8 9 10 11 12];
      |    Select3_PortWidth=12;
      | end
      | power_initmask();
      mask Help:
      | The output pulses are a vector (with values=0 or 1). Depending on the selected "Generator Mode", the output vector contains:
      | For a 1-arm  bridge: Two pulses. Pulse 1 is for the upper switch and pulse 2 is for the lower switch.
      | For a 2-arm  bridge: Four pulses. Pulses 1 and 3 are respectively for the upper switches of the first and second arm. Pulses 2 and 4 are for the lower switches.
      | For a 3-arm  bridge: Six pulses. Pulses 1,3 and 5 are respectively for the upper switches of the first,second and third arm. Pulses 2,4 and 6 are for the lower switches.
      | For double 3-arm bridges: Twelve pulses.The first six pulses (pulses 1 to 6) must be sent to the first 3-arm bridge and the last six (pulses 7 to 12) to the second 3-arm bridge.
      | 
      | By selecting "Internal generation" you can can control the modulation index m, frequency and phase of the output voltage  from the internal parameters (m, Freq and Phase). Otherwise, external signals are used for pulse generation. The width of the input vector must be 1 for single phase bridges ( 1-arm or 2-arm)  and 3 for 3-phase bridges  (single or double bridge).
      mask TypeOptions GeneratorMode: 1-arm  bridge (2 pulses) | 2-arm  bridge (4 pulses) | 3-arm  bridge (6 pulses) | Double 3-arm  bridges (12 pulses)
      mask Callback Internal: powericon('psbcallbacks',gcb,'Discrete PWM Generator',[]);
  MI Controller : Subsystem
  Subsystem1 : Subsystem
  Unit Delay4 : UnitDelay  SampleTime=20e-6  HasFrameUpgradeWarning=on
  C : PMIOPort  Side=Left
  B : PMIOPort  Port=2  Side=Left
  A : PMIOPort  Port=3  Side=Left
  VL : Outport  VectorParamsAs1DForOutWhenUnconnected=off
  Vp : Outport  Port=2  VectorParamsAs1DForOutWhenUnconnected=off
  Pulses : Outport  Port=3  VectorParamsAs1DForOutWhenUnconnected=off
  wires:
  Unit Delay4/1 -> Pulses/1
  Discrete PWM Generator1/1(Pulses) -> Unit Delay4/1
  MI Controller/1(Vabc_inv) -> Discrete PWM Generator1/1(Uref)
  Subsystem1/1(Vph) -> MI Controller/1(Vabc)
  Subsystem1/2(VL-L) -> VL/1
  Subsystem1/3(Vph_rms) -> Vp/1
  connections:
  A/RConn1 -- Subsystem1/LConn1
  B/RConn1 -- Subsystem1/LConn2
  C/RConn1 -- Subsystem1/LConn3

== system WindPrototipeN/Дом 1/DC//DC ПРЕОБРАЗОВАТЕЛЬ ВЭУ/Chopper ==
  Duty Cycle : Inport
  Average-value armature voltage : Fcn  Expr=u(1)*u(2)
  Average-value source current : Fcn  Expr=u(1)*u(2)
  Controlled Current Source : powerlib/Electrical Sources/Controlled Current Source  Initialize=on  Source_Type=AC  Amplitude=0  Phase=0  Frequency=0  Measurements=None
      settings: SourceProductName=Simscape Electrical
  Controlled Voltage Source : powerlib/Electrical Sources/Controlled Voltage Source  Initialize=on  Source_Type=AC  Amplitude=0  Phase=0  Frequency=0  Measurements=None
      settings: SourceProductName=Simscape Electrical
  Current Measurement : powerlib/Measurements/Current Measurement  Tag=PoWeRsYsTeMmEaSuReMeNt  PhasorSimulation=off  OutputType=Magnitude  PSBequivalent=0
      settings: SourceProductName=Simscape Electrical
  Memory : Memory
  Memory1 : Memory
  Mux : Mux  Inputs=2
  Mux1 : Mux  Inputs=2
  Selector : Selector  InputPortWidth=2  IndexOptions=Index vector (dialog)  Indices=[1]  OutputSizes=1
  Voltage Measurement1 : powerlib/Measurements/Voltage Measurement  Tag=PoWeRsYsTeMmEaSuReMeNt  PhasorSimulation=off  OutputType=Magnitude  PSBequivalent=0
      settings: SourceProductName=Simscape Electrical
  A : PMIOPort  Side=Right
  + : PMIOPort  Port=2  Side=Left
  - : PMIOPort  Port=3  Side=Left
  wires:
  Memory/1 -> Controlled Voltage Source/1
  Average-value armature voltage/1 -> Memory/1
  Mux/1 -> Average-value armature voltage/1
  Voltage Measurement1/1 -> Mux/2
  Duty Cycle/1 -> Selector/1
  Mux1/1 -> Average-value source current/1
  Current Measurement/1 -> Mux1/2
  Average-value source current/1 -> Memory1/1
  Memory1/1 -> Controlled Current Source/1
  Selector/1 -> Mux/1, Mux1/1
  connections:
  Voltage Measurement1/LConn2 -- Controlled Current Source/RConn1 -- -/RConn1 -- Controlled Voltage Source/LConn1
  Controlled Current Source/LConn1 -- Voltage Measurement1/LConn1 -- +/RConn1
  Controlled Voltage Source/RConn1 -- Current Measurement/LConn1
  A/RConn1 -- Current Measurement/RConn1

== system WindPrototipeN/Дом 1/DC//DC ПРЕОБРАЗОВАТЕЛЬ ВЭУ/Current controller DISCRETE1 ==
  UBus : Inport
  Uref : Inport  Port=2
  Ctrl sat. : Saturate  UpperLimit=0.95  LowerLimit=-0.95
  Discrete-Time Integrator : DiscreteIntegrator  IntegratorMethod=Integration: Trapezoidal  SampleTime=Ts  LimitOutput=on  UpperSaturationLimit=0.95  LowerSaturationLimit=-0.95  ICPrevOutput=DiscIntNeverNeededParam  ICPrevScaledInput=DiscIntNeverNeededParam
  Integral gain : Gain  Gain=Ki  SaturateOnIntegerOverflow=on  OutDataTypeStr=Inherit: Same as input  ParamDataTypeStr=Inherit: Same as input
  Proportional gain : Gain  Gain=Kp  SaturateOnIntegerOverflow=on  OutDataTypeStr=Inherit: Same as input  ParamDataTypeStr=Inherit: Same as input
  Sum1 : Sum  Inputs=+-  SaturateOnIntegerOverflow=on  InputSameDT=on  OutDataTypeStr=Inherit: Same as first input
  Sum2 : Sum  SaturateOnIntegerOverflow=on  InputSameDT=on  OutDataTypeStr=Inherit: Same as first input
  Ec : Outport  InitialOutput=0  VectorParamsAs1DForOutWhenUnconnected=off
  wires:
  Proportional gain/1 -> Sum2/1
  Integral gain/1 -> Discrete-Time Integrator/1
  Sum1/1 -> Integral gain/1, Proportional gain/1
  UBus/1 -> Sum1/1
  Uref/1 -> Sum1/2
  Discrete-Time Integrator/1 -> Sum2/2
  Sum2/1 -> Ctrl sat./1
  Ctrl sat./1 -> Ec/1

== system WindPrototipeN/Дом 1/DC//DC ПРЕОБРАЗОВАТЕЛЬ ВЭУ/Current controller DISCRETE2 ==
  Pref : Inport
  Ppv : Inport  Port=2
  Ctrl sat. : Saturate  UpperLimit=0.95  LowerLimit=-0.95
  Discrete-Time Integrator : DiscreteIntegrator  IntegratorMethod=Integration: Trapezoidal  SampleTime=Ts  LimitOutput=on  UpperSaturationLimit=0.95  LowerSaturationLimit=-0.95  ICPrevOutput=DiscIntNeverNeededParam  ICPrevScaledInput=DiscIntNeverNeededParam
  Integral gain : Gain  Gain=Ki  SaturateOnIntegerOverflow=on  OutDataTypeStr=Inherit: Same as input  ParamDataTypeStr=Inherit: Same as input
  Proportional gain : Gain  Gain=Kp  SaturateOnIntegerOverflow=on  OutDataTypeStr=Inherit: Same as input  ParamDataTypeStr=Inherit: Same as input
  Sum1 : Sum  Inputs=+-  SaturateOnIntegerOverflow=on  InputSameDT=on  OutDataTypeStr=Inherit: Same as first input
  Sum2 : Sum  SaturateOnIntegerOverflow=on  InputSameDT=on  OutDataTypeStr=Inherit: Same as first input
  Delta Ec : Outport  InitialOutput=0  VectorParamsAs1DForOutWhenUnconnected=off
  wires:
  Ctrl sat./1 -> Delta Ec/1
  Sum2/1 -> Ctrl sat./1
  Discrete-Time Integrator/1 -> Sum2/2
  Ppv/1 -> Sum1/2
  Pref/1 -> Sum1/1
  Sum1/1 -> Proportional gain/1, Integral gain/1
  Integral gain/1 -> Discrete-Time Integrator/1
  Proportional gain/1 -> Sum2/1

== system WindPrototipeN/Дом 1/DC//DC ПРЕОБРАЗОВАТЕЛЬ ВЭУ/Duty Cycles ==
  Ec : Inport
  Add : Sum  Inputs=+-
  Bus Creator2 : BusCreator  Inputs=2
  Constant : Constant
  Duty Cycle : Fcn  Expr=0.5*(u[1]+1)
  dc : Outport  VectorParamsAs1DForOutWhenUnconnected=off
  wires:
  Duty Cycle/1 -> Add/2, Bus Creator2/1  "IGBT I"
  Add/1 -> Bus Creator2/2  "IGBT 2"
  Constant/1 -> Add/1
  Ec/1 -> Duty Cycle/1
  Bus Creator2/1 -> dc/1

== system WindPrototipeN/Дом 1/DC//DC ПРЕОБРАЗОВАТЕЛЬ ВЭУ/Timer ==
  Clock : Clock
  Derivative : Derivative
  Hit Crossing : HitCross  ShowOutputPort=off
  Look-Up Table : Lookup  InputValues=tv  Table=opv  SaturateOnIntegerOverflow=on
  Out : Outport  VectorParamsAs1DForOutWhenUnconnected=off
  wires:
  Clock/1 -> Look-Up Table/1
  Look-Up Table/1 -> Out/1, Derivative/1
  Derivative/1 -> Hit Crossing/1

== system WindPrototipeN/Дом 1/DC//DC ПРЕОБРАЗОВАТЕЛЬ СП/Chopper ==
  Duty Cycle : Inport
  Average-value armature voltage : Fcn  Expr=u(1)*u(2)
  Average-value source current : Fcn  Expr=u(1)*u(2)
  Controlled Current Source : powerlib/Electrical Sources/Controlled Current Source  Initialize=on  Source_Type=AC  Amplitude=0  Phase=0  Frequency=0  Measurements=None
      settings: SourceProductName=Simscape Electrical
  Controlled Voltage Source : powerlib/Electrical Sources/Controlled Voltage Source  Initialize=on  Source_Type=AC  Amplitude=0  Phase=0  Frequency=0  Measurements=None
      settings: SourceProductName=Simscape Electrical
  Current Measurement : powerlib/Measurements/Current Measurement  Tag=PoWeRsYsTeMmEaSuReMeNt  PhasorSimulation=off  OutputType=Magnitude  PSBequivalent=0
      settings: SourceProductName=Simscape Electrical
  Memory : Memory
  Memory1 : Memory
  Mux : Mux  Inputs=2
  Mux1 : Mux  Inputs=2
  Selector : Selector  InputPortWidth=2  IndexOptions=Index vector (dialog)  Indices=[1]  OutputSizes=1
  Voltage Measurement1 : powerlib/Measurements/Voltage Measurement  Tag=PoWeRsYsTeMmEaSuReMeNt  PhasorSimulation=off  OutputType=Magnitude  PSBequivalent=0
      settings: SourceProductName=Simscape Electrical
  A : PMIOPort  Side=Right
  + : PMIOPort  Port=2  Side=Left
  - : PMIOPort  Port=3  Side=Left
  wires:
  Memory/1 -> Controlled Voltage Source/1
  Average-value armature voltage/1 -> Memory/1
  Mux/1 -> Average-value armature voltage/1
  Voltage Measurement1/1 -> Mux/2
  Duty Cycle/1 -> Selector/1
  Mux1/1 -> Average-value source current/1
  Current Measurement/1 -> Mux1/2
  Average-value source current/1 -> Memory1/1
  Memory1/1 -> Controlled Current Source/1
  Selector/1 -> Mux/1, Mux1/1
  connections:
  Voltage Measurement1/LConn2 -- Controlled Current Source/RConn1 -- -/RConn1 -- Controlled Voltage Source/LConn1
  Controlled Current Source/LConn1 -- Voltage Measurement1/LConn1 -- +/RConn1
  Controlled Voltage Source/RConn1 -- Current Measurement/LConn1
  A/RConn1 -- Current Measurement/RConn1

== system WindPrototipeN/Дом 1/DC//DC ПРЕОБРАЗОВАТЕЛЬ СП/Current controller DISCRETE1 ==
  UBus : Inport
  Uref : Inport  Port=2
  Ctrl sat. : Saturate  UpperLimit=0.95  LowerLimit=-0.95
  Discrete-Time Integrator : DiscreteIntegrator  IntegratorMethod=Integration: Trapezoidal  SampleTime=Ts  LimitOutput=on  UpperSaturationLimit=0.95  LowerSaturationLimit=-0.95  ICPrevOutput=DiscIntNeverNeededParam  ICPrevScaledInput=DiscIntNeverNeededParam
  Integral gain : Gain  Gain=Ki  SaturateOnIntegerOverflow=on  OutDataTypeStr=Inherit: Same as input  ParamDataTypeStr=Inherit: Same as input
  Proportional gain : Gain  Gain=Kp  SaturateOnIntegerOverflow=on  OutDataTypeStr=Inherit: Same as input  ParamDataTypeStr=Inherit: Same as input
  Sum1 : Sum  Inputs=+-  SaturateOnIntegerOverflow=on  InputSameDT=on  OutDataTypeStr=Inherit: Same as first input
  Sum2 : Sum  SaturateOnIntegerOverflow=on  InputSameDT=on  OutDataTypeStr=Inherit: Same as first input
  Ec : Outport  InitialOutput=0  VectorParamsAs1DForOutWhenUnconnected=off
  wires:
  Proportional gain/1 -> Sum2/1
  Integral gain/1 -> Discrete-Time Integrator/1
  Sum1/1 -> Integral gain/1, Proportional gain/1
  UBus/1 -> Sum1/1
  Uref/1 -> Sum1/2
  Discrete-Time Integrator/1 -> Sum2/2
  Sum2/1 -> Ctrl sat./1
  Ctrl sat./1 -> Ec/1
